simulink model "mrefrobotarm_previous_y_previous_u_previous_ref_cex_3"  (R2018b)
settings: Solver=FixedStepAuto  StartTime=0.0  StopTime=20  RelTol=1e-3  AbsTol=1e-6
undefined symbols (not defined in the file or in its folder): cc, options
libraries: neural x396, simulink x2
(part 11 of 15)

== system mrefrobotarm_previous_y_previous_u_previous_ref_cex_3/cex_m4_10_cl/Layer 3/Delays 1 ==
  "p{3}" : Inport  PortDimensions=30
      mask Display: e = 0.06;c1 = [120 230 180]/255;c2 = ([120 230 180]+0)/(256+128);c3 = ([120 230 180]+128)/(256+128);patch([0 1 1 0],[0 0 1 1],c1);patch([0 1 1 1-e 1-e 0+e],[0 0 1 1-e 0+e 0+e],c2);patch([0 0 1 1-e 0+e 0+e],[0 1 1 1-e 1-e 0+e],c3);plot([0 1 1 0 0],[0 0 1 1 0]);
  mux : Mux  Inputs=1
      mask Display: e = 0.06;c1 = [120 150 230]/255;c2 = ([120 150 230]+0)/383;c3 = ([120 150 230]+128)/383;patch([0 1 1 0],[0 0 1 1],c1);patch([0 1 1 1-e 1-e 0+e],[0 0 1 1-e 0+e 0+e],c2);patch([0 0 1 1-e 0+e 0+e],[0 1 1 1-e 1-e 0+e],c3);plot([0 1 1 0 0],[0 0 1 1 0]);disp('Mux')
  "pd{3,2}" : Outport
      mask Display: e = 0.06;c1 = [120 230 180]/255;c2 = ([120 230 180]+0)/(256+128);c3 = ([120 230 180]+128)/(256+128);patch([0 1 1 0],[0 0 1 1],c1);patch([0 1 1 1-e 1-e 0+e],[0 0 1 1-e 0+e 0+e],c2);patch([0 0 1 1-e 0+e 0+e],[0 1 1 1-e 1-e 0+e],c3);plot([0 1 1 0 0],[0 0 1 1 0]);
  wires:
  "p{3}"/1 -> mux/1
  mux/1 -> "pd{3,2}"/1

== system mrefrobotarm_previous_y_previous_u_previous_ref_cex_3/cex_m4_10_cl/Layer 3/LW{3,2} ==
  "ad{3,2}" : Inport  PortDimensions=30
      mask Display: e = 0.06;c1 = [120 230 180]/255;c2 = ([120 230 180]+0)/(256+128);c3 = ([120 230 180]+128)/(256+128);patch([0 1 1 0],[0 0 1 1],c1);patch([0 1 1 1-e 1-e 0+e],[0 0 1 1-e 0+e 0+e],c2);patch([0 0 1 1-e 0+e 0+e],[0 1 1 1-e 1-e 0+e],c3);plot([0 1 1 0 0],[0 0 1 1 0]);
  "IW{3,2}(1,:)'" : Constant  Value=[-0.022914673180611945524365324899918050505220890045166015625;-0.22416800997145325258230741383158601820468902587890625;0.42578222016399902560834789255750365555286407470703125;-0.1418372366772850667882011066467384807765483856201171875;0.06806813579219629650740586157553480006754398345947265625;-0.26711253758643660471960856739315204322338104248046875;-0.288746492548126509891659452478052116930484771728515625;0.1568382571083110355036893679425702430307865142822265625;-0.1365854357814726416364692340721376240253448486328125;0.86307011627554930388583898093202151358127593994140625;0.314580357392832132834570302293286658823490142822265625;0.056739431746669545530981082492871792055666446685791015625;-0.036816877975223871732879388218862004578113555908203125;-0.04310990977375095400958571190130896866321563720703125;0.1941188152854624870968791583436541259288787841796875;0.2071271857104373947944253586683771573007106781005859375;-0.1944372739173033381998578761340468190610408782958984375;0.47407063712269736921456342315650545060634613037109375;-0.0147826682194927526425853869795901118777692317962646484375;0.01471526546516824067445394774722444708459079265594482421875;0.2010572904622072998304105340139358304440975189208984375;-0.004037117964215650688097891674033235176466405391693115234375;0.254448141541254890807266519914264790713787078857421875;-0.343286635301220222071805210362072102725505828857421875;-0.06292101207340337898354931667199707590043544769287109375;-0.034537508248897015594724990705799427814781665802001953125;0.2287289337043199310972596549618174321949481964111328125;0.472236103182088806651250934010022319853305816650390625;-0.142786618432387102384240051833330653607845306396484375;0.45708708531073305447733901019091717898845672607421875]
      mask Display: e = 0.06;c1 = [120 150 230]/255;c2 = ([120 150 230]+0)/383;c3 = ([120 150 230]+128)/383;patch([0 1 1 0],[0 0 1 1],c1);patch([0 1 1 1-e 1-e 0+e],[0 0 1 1-e 0+e 0+e],c2);patch([0 0 1 1-e 0+e 0+e],[0 1 1 1-e 1-e 0+e],c3);plot([0 1 1 0 0],[0 0 1 1 0]);disp('weights');
  Mux : Mux  Inputs=1
      mask Display: e = 0.06;c1 = [120 150 230]/255;c2 = ([120 150 230]+0)/383;c3 = ([120 150 230]+128)/383;patch([0 1 1 0],[0 0 1 1],c1);patch([0 1 1 1-e 1-e 0+e],[0 0 1 1-e 0+e 0+e],c2);patch([0 0 1 1-e 0+e 0+e],[0 1 1 1-e 1-e 0+e],c3);plot([0 1 1 0 0],[0 0 1 1 0]);disp('Mux');
  dotprod1 : neural/Weight Functions/dotprod
  "lz{3,2}" : Outport
      mask Display: e = 0.06;c1 = [120 230 180]/255;c2 = ([120 230 180]+0)/(256+128);c3 = ([120 230 180]+128)/(256+128);patch([0 1 1 0],[0 0 1 1],c1);patch([0 1 1 1-e 1-e 0+e],[0 0 1 1-e 0+e 0+e],c2);patch([0 0 1 1-e 0+e 0+e],[0 1 1 1-e 1-e 0+e],c3);plot([0 1 1 0 0],[0 0 1 1 0]);
  wires:
  "IW{3,2}(1,:)'"/1 -> dotprod1/1
  "ad{3,2}"/1 -> dotprod1/2
  dotprod1/1 -> Mux/1
  Mux/1 -> "lz{3,2}"/1

== system mrefrobotarm_previous_y_previous_u_previous_ref_cex_3/cex_m5_50/Layer 1/Delays 1 ==
  "p{1}" : Inport  PortDimensions=10
      mask Display: e = 0.06;c1 = [120 230 180]/255;c2 = ([120 230 180]+0)/(256+128);c3 = ([120 230 180]+128)/(256+128);patch([0 1 1 0],[0 0 1 1],c1);patch([0 1 1 1-e 1-e 0+e],[0 0 1 1-e 0+e 0+e],c2);patch([0 0 1 1-e 0+e 0+e],[0 1 1 1-e 1-e 0+e],c3);plot([0 1 1 0 0],[0 0 1 1 0]);
  mux : Mux  Inputs=1
      mask Display: e = 0.06;c1 = [120 150 230]/255;c2 = ([120 150 230]+0)/383;c3 = ([120 150 230]+128)/383;patch([0 1 1 0],[0 0 1 1],c1);patch([0 1 1 1-e 1-e 0+e],[0 0 1 1-e 0+e 0+e],c2);patch([0 0 1 1-e 0+e 0+e],[0 1 1 1-e 1-e 0+e],c3);plot([0 1 1 0 0],[0 0 1 1 0]);disp('Mux')
  "pd{1,1}" : Outport
      mask Display: e = 0.06;c1 = [120 230 180]/255;c2 = ([120 230 180]+0)/(256+128);c3 = ([120 230 180]+128)/(256+128);patch([0 1 1 0],[0 0 1 1],c1);patch([0 1 1 1-e 1-e 0+e],[0 0 1 1-e 0+e 0+e],c2);patch([0 0 1 1-e 0+e 0+e],[0 1 1 1-e 1-e 0+e],c3);plot([0 1 1 0 0],[0 0 1 1 0]);
  wires:
  "p{1}"/1 -> mux/1
  mux/1 -> "pd{1,1}"/1

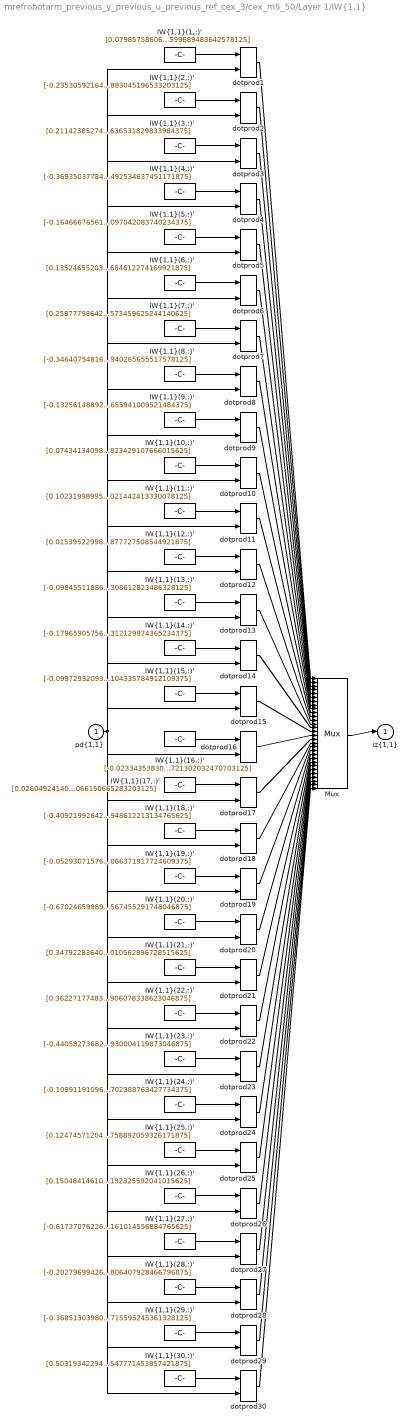
== system mrefrobotarm_previous_y_previous_u_previous_ref_cex_3/cex_m5_50/Layer 1/IW{1,1} ==
  "pd{1,1}" : Inport  PortDimensions=10
      mask Display: e = 0.06;c1 = [120 230 180]/255;c2 = ([120 230 180]+0)/(256+128);c3 = ([120 230 180]+128)/(256+128);patch([0 1 1 0],[0 0 1 1],c1);patch([0 1 1 1-e 1-e 0+e],[0 0 1 1-e 0+e 0+e],c2);patch([0 0 1 1-e 0+e 0+e],[0 1 1 1-e 1-e 0+e],c3);plot([0 1 1 0 0],[0 0 1 1 0]);
  "IW{1,1}(1,:)'" : Constant  Value=[0.079857586064122687563582303482689894735813140869140625;-0.017723095364553236030769056696954066865146160125732421875;-0.056548854768613217303130369373320718295872211456298828125;-0.10470870115022480606459254204310127533972263336181640625;-0.11145776410343340157016456259952974505722522735595703125;-0.040973627042265363396023047926064464263617992401123046875;-0.2352542960460574927861188143651816062629222869873046875;0.074050472634338226907146918165381066501140594482421875;-0.1791921386348343248062775501239229924976825714111328125;0.1353912225675833191917973863382940180599689483642578125]
      mask Display: e = 0.06;c1 = [120 150 230]/255;c2 = ([120 150 230]+0)/383;c3 = ([120 150 230]+128)/383;patch([0 1 1 0],[0 0 1 1],c1);patch([0 1 1 1-e 1-e 0+e],[0 0 1 1-e 0+e 0+e],c2);patch([0 0 1 1-e 0+e 0+e],[0 1 1 1-e 1-e 0+e],c3);plot([0 1 1 0 0],[0 0 1 1 0]);disp('Weights');
  "IW{1,1}(10,:)'" : Constant  Value=[0.0743413409874611463834526148275472223758697509765625;0.164396607140263883994890647954889573156833648681640625;-0.143955487553599936756398847137461416423320770263671875;-0.0721315099709873563949003028028528206050395965576171875;0.1556391323832038986463288665618165396153926849365234375;-0.15582294381245664904866998767829500138759613037109375;0.0193247847981503732828212349659224855713546276092529296875;-0.1039680088534420676626979229695280082523822784423828125;0.08318682925150173990136437396358815021812915802001953125;-0.2231496668480378586796319950735778547823429107666015625]
      mask Display: e = 0.06;c1 = [120 150 230]/255;c2 = ([120 150 230]+0)/383;c3 = ([120 150 230]+128)/383;patch([0 1 1 0],[0 0 1 1],c1);patch([0 1 1 1-e 1-e 0+e],[0 0 1 1-e 0+e 0+e],c2);patch([0 0 1 1-e 0+e 0+e],[0 1 1 1-e 1-e 0+e],c3);plot([0 1 1 0 0],[0 0 1 1 0]);disp('Weights');
  "IW{1,1}(11,:)'" : Constant  Value=[0.102319989954805679044369526309310458600521087646484375;-0.1217472670747620500097951889983960427343845367431640625;0.022250510998612631208271039895407739095389842987060546875;-0.0865197557599649280657416738904430530965328216552734375;0.047157973574144917972006396666984073817729949951171875;0.166311308504842270128420977925998158752918243408203125;-0.07692919866478746537818977913048001937568187713623046875;0.1289101580164291604990722817092319019138813018798828125;-0.03712492046256300748385825727382325567305088043212890625;0.0862830620540880055546750782013987191021442413330078125]
      mask Display: e = 0.06;c1 = [120 150 230]/255;c2 = ([120 150 230]+0)/383;c3 = ([120 150 230]+128)/383;patch([0 1 1 0],[0 0 1 1],c1);patch([0 1 1 1-e 1-e 0+e],[0 0 1 1-e 0+e 0+e],c2);patch([0 0 1 1-e 0+e 0+e],[0 1 1 1-e 1-e 0+e],c3);plot([0 1 1 0 0],[0 0 1 1 0]);disp('Weights');
  "IW{1,1}(12,:)'" : Constant  Value=[0.0153952299864565760045831410707251052372157573699951171875;-0.29382621968364486253477707577985711395740509033203125;0.15069864020460455034111646455130539834499359130859375;0.129272775534195083491084687921102158725261688232421875;-0.00719280555420370899810666998064334620721638202667236328125;0.017590441101808795831829002054291777312755584716796875;-0.1455726439346946843311769725914928130805492401123046875;-0.1131091311033599888791201237836503423750400543212890625;0.144361291612564779374139334322535432875156402587890625;-0.1039940199905408924063721087804879061877727508544921875]
      mask Display: e = 0.06;c1 = [120 150 230]/255;c2 = ([120 150 230]+0)/383;c3 = ([120 150 230]+128)/383;patch([0 1 1 0],[0 0 1 1],c1);patch([0 1 1 1-e 1-e 0+e],[0 0 1 1-e 0+e 0+e],c2);patch([0 0 1 1-e 0+e 0+e],[0 1 1 1-e 1-e 0+e],c3);plot([0 1 1 0 0],[0 0 1 1 0]);disp('Weights');
  "IW{1,1}(13,:)'" : Constant  Value=[-0.09845511886806544710193378477924852631986141204833984375;0.09093880387205426074626046784032951109111309051513671875;-0.00807145029070374143975730163447224185802042484283447265625;0.1579263851539709495597207933315075933933258056640625;-0.0894690058866917381497074757135123945772647857666015625;-0.0062623475836107826697496392398534226231276988983154296875;0.06411970043190341750349858784829848445951938629150390625;-0.11454387947590256857655077737945248372852802276611328125;-0.16589537965291556442792852976708672940731048583984375;0.197603240212231856531843732227571308612823486328125]
      mask Display: e = 0.06;c1 = [120 150 230]/255;c2 = ([120 150 230]+0)/383;c3 = ([120 150 230]+128)/383;patch([0 1 1 0],[0 0 1 1],c1);patch([0 1 1 1-e 1-e 0+e],[0 0 1 1-e 0+e 0+e],c2);patch([0 0 1 1-e 0+e 0+e],[0 1 1 1-e 1-e 0+e],c3);plot([0 1 1 0 0],[0 0 1 1 0]);disp('Weights');
  "IW{1,1}(14,:)'" : Constant  Value=[-0.1796590575681936419183415409861481748521327972412109375;0.004065668616646420270577255706712094251997768878936767578125;0.1660524217557300674652509542283951304852962493896484375;-0.018752259357130311723249604938246193341910839080810546875;-0.0166360990303930332545601089577758102677762508392333984375;0.156250719589604736281529540065093897283077239990234375;0.143670141139804530272527927081682719290256500244140625;0.197765834991741107362628326882258988916873931884765625;-0.115318383987298600512616530977538786828517913818359375;0.06920828841457514479795776196624501608312129974365234375]
      mask Display: e = 0.06;c1 = [120 150 230]/255;c2 = ([120 150 230]+0)/383;c3 = ([120 150 230]+128)/383;patch([0 1 1 0],[0 0 1 1],c1);patch([0 1 1 1-e 1-e 0+e],[0 0 1 1-e 0+e 0+e],c2);patch([0 0 1 1-e 0+e 0+e],[0 1 1 1-e 1-e 0+e],c3);plot([0 1 1 0 0],[0 0 1 1 0]);disp('Weights');
  "IW{1,1}(15,:)'" : Constant  Value=[-0.0997293209396606095129556024403427727520465850830078125;-0.220637160043276825405200725072063505649566650390625;-0.00148221978238747219801252352766596231958828866481781005859375;-0.2518385145644688183352855048724450170993804931640625;-0.226371647407521858763601585451397113502025604248046875;-0.183592461943430762527640354164759628474712371826171875;-0.0281470738205235916640223337026327499188482761383056640625;-0.183673166456358061271458836927195079624652862548828125;0.03735748593921994764599503469071350991725921630859375;-0.083966000578261590359119281856692396104335784912109375]
      mask Display: e = 0.06;c1 = [120 150 230]/255;c2 = ([120 150 230]+0)/383;c3 = ([120 150 230]+128)/383;patch([0 1 1 0],[0 0 1 1],c1);patch([0 1 1 1-e 1-e 0+e],[0 0 1 1-e 0+e 0+e],c2);patch([0 0 1 1-e 0+e 0+e],[0 1 1 1-e 1-e 0+e],c3);plot([0 1 1 0 0],[0 0 1 1 0]);disp('Weights');
  "IW{1,1}(16,:)'" : Constant  Value=[-0.023343538302298010023161367598731885664165019989013671875;0.207808437401322265714043169282376766204833984375;0.19767903767718764118654917183448560535907745361328125;0.08721736450330919154794173664413392543792724609375;-0.1026675757733719607234235127179999835789203643798828125;0.1893806324687653253047159296329482458531856536865234375;0.157181246537321739342729642885387875139713287353515625;-0.0762455615664333341552350020720041356980800628662109375;0.1511383886935200038248439113885979168117046356201171875;-0.032936019457746275318488216043988359160721302032470703125]
      mask Display: e = 0.06;c1 = [120 150 230]/255;c2 = ([120 150 230]+0)/383;c3 = ([120 150 230]+128)/383;patch([0 1 1 0],[0 0 1 1],c1);patch([0 1 1 1-e 1-e 0+e],[0 0 1 1-e 0+e 0+e],c2);patch([0 0 1 1-e 0+e 0+e],[0 1 1 1-e 1-e 0+e],c3);plot([0 1 1 0 0],[0 0 1 1 0]);disp('Weights');
  "IW{1,1}(17,:)'" : Constant  Value=[0.026049241400837468141116204378704424016177654266357421875;-0.032936276559719333822950915191540843807160854339599609375;-0.09167093550109205180032034832038334570825099945068359375;-0.1285074909294273981519296512487926520407199859619140625;0.078280680856052831106950407047406770288944244384765625;0.035046276117616514955699358324636705219745635986328125;0.04575276258096482029369411748120910488069057464599609375;-0.1455865211885374044253893544009770266711711883544921875;-0.16108537419119872691197770109283737838268280029296875;-0.25221969637927810214961255041998811066150665283203125]
      mask Display: e = 0.06;c1 = [120 150 230]/255;c2 = ([120 150 230]+0)/383;c3 = ([120 150 230]+128)/383;patch([0 1 1 0],[0 0 1 1],c1);patch([0 1 1 1-e 1-e 0+e],[0 0 1 1-e 0+e 0+e],c2);patch([0 0 1 1-e 0+e 0+e],[0 1 1 1-e 1-e 0+e],c3);plot([0 1 1 0 0],[0 0 1 1 0]);disp('Weights');
  "IW{1,1}(18,:)'" : Constant  Value=[-0.409219926426756586135269344595144502818584442138671875;0.0785959772336427830996541388230980373919010162353515625;-0.150796017332621434814399208335089497268199920654296875;0.054714100522777205093394314872057293541729450225830078125;-0.197699818473965283072146803533541969954967498779296875;0.079927612600015407462450411912868730723857879638671875;0.0100629098409829621785238629172454238869249820709228515625;-0.2085223358752021083351024799412698484957218170166015625;0.1160915267315043575280242293956689536571502685546875;-0.039902292098272375275858081522528664208948612213134765625]
      mask Display: e = 0.06;c1 = [120 150 230]/255;c2 = ([120 150 230]+0)/383;c3 = ([120 150 230]+128)/383;patch([0 1 1 0],[0 0 1 1],c1);patch([0 1 1 1-e 1-e 0+e],[0 0 1 1-e 0+e 0+e],c2);patch([0 0 1 1-e 0+e 0+e],[0 1 1 1-e 1-e 0+e],c3);plot([0 1 1 0 0],[0 0 1 1 0]);disp('Weights');
  "IW{1,1}(19,:)'" : Constant  Value=[-0.05293071576668927080699944553998648189008235931396484375;-0.0784315336245811345339262743436847813427448272705078125;0.052396564711746758391530676135516841895878314971923828125;-0.045966369293603072387899288742119097150862216949462890625;0.1996321210973512894071291157160885632038116455078125;-0.047923892413621015096136801503234892152249813079833984375;0.250968980826343390777566355609451420605182647705078125;0.0226665665494998093409950712384670623578131198883056640625;-0.1273645483236649778024940360410255379974842071533203125;-0.0881084613766523749855963387744850479066371917724609375]
      mask Display: e = 0.06;c1 = [120 150 230]/255;c2 = ([120 150 230]+0)/383;c3 = ([120 150 230]+128)/383;patch([0 1 1 0],[0 0 1 1],c1);patch([0 1 1 1-e 1-e 0+e],[0 0 1 1-e 0+e 0+e],c2);patch([0 0 1 1-e 0+e 0+e],[0 1 1 1-e 1-e 0+e],c3);plot([0 1 1 0 0],[0 0 1 1 0]);disp('Weights');
  "IW{1,1}(2,:)'" : Constant  Value=[-0.2353059216442040246786149282343103550374507904052734375;-0.37789763749456184438457739815930835902690887451171875;0.214493078021647687325668130142730660736560821533203125;0.130691057428845069932066280671278946101665496826171875;0.192062118999956565890130377738387323915958404541015625;0.09267188455379683775792187816477962769567966461181640625;0.04144170290809519319186193797577288933098316192626953125;-0.016488872173757489203449466685924562625586986541748046875;-0.411465202425676135344900785639765672385692596435546875;0.1802654075409109435401688870115322060883045196533203125]
      mask Display: e = 0.06;c1 = [120 150 230]/255;c2 = ([120 150 230]+0)/383;c3 = ([120 150 230]+128)/383;patch([0 1 1 0],[0 0 1 1],c1);patch([0 1 1 1-e 1-e 0+e],[0 0 1 1-e 0+e 0+e],c2);patch([0 0 1 1-e 0+e 0+e],[0 1 1 1-e 1-e 0+e],c3);plot([0 1 1 0 0],[0 0 1 1 0]);disp('Weights');
  "IW{1,1}(20,:)'" : Constant  Value=[-0.670246599899003481226600342779420316219329833984375;0.54023279823907544017203008479555137455463409423828125;-0.132643633303448360560850005640531890094280242919921875;-0.08573477507453254597979963591569685377180576324462890625;-0.05214787663669749606665249075376777909696102142333984375;-0.24868608156944926879106105843675322830677032470703125;-0.0708532779744801555210642618476413190364837646484375;-0.1612321158738975468427412351957173086702823638916015625;-0.377010414829936857383785309139057062566280364990234375;-0.326354942562080363455123688254388980567455291748046875]
      mask Display: e = 0.06;c1 = [120 150 230]/255;c2 = ([120 150 230]+0)/383;c3 = ([120 150 230]+128)/383;patch([0 1 1 0],[0 0 1 1],c1);patch([0 1 1 1-e 1-e 0+e],[0 0 1 1-e 0+e 0+e],c2);patch([0 0 1 1-e 0+e 0+e],[0 1 1 1-e 1-e 0+e],c3);plot([0 1 1 0 0],[0 0 1 1 0]);disp('Weights');
  "IW{1,1}(21,:)'" : Constant  Value=[0.34792283640337806627229610967333428561687469482421875;0.052295351768964971894693150034072459675371646881103515625;0.215517399724929281656926605137414298951625823974609375;-0.10110471240800637804380102124923723749816417694091796875;-0.1307353664929510606018681073692278005182743072509765625;0.152266018278392090135042735710158012807369232177734375;-0.149298402696842857917403080136864446103572845458984375;0.044436751362071459647840043771793716587126255035400390625;0.256340040153919812571103875598055310547351837158203125;0.05083490551971847626333556036115624010562896728515625]
      mask Display: e = 0.06;c1 = [120 150 230]/255;c2 = ([120 150 230]+0)/383;c3 = ([120 150 230]+128)/383;patch([0 1 1 0],[0 0 1 1],c1);patch([0 1 1 1-e 1-e 0+e],[0 0 1 1-e 0+e 0+e],c2);patch([0 0 1 1-e 0+e 0+e],[0 1 1 1-e 1-e 0+e],c3);plot([0 1 1 0 0],[0 0 1 1 0]);disp('Weights');
  "IW{1,1}(22,:)'" : Constant  Value=[0.362271774839149018898609710959135554730892181396484375;-0.1319520713686885837745421667932532727718353271484375;-0.1014321707030214347877716818402404896914958953857421875;-0.09152058110484677377893802940889145247638225555419921875;-0.0042955190046048523366817306623488548211753368377685546875;0.01111324222692758496855436334271871601231396198272705078125;0.1775136539958918902026852038034121505916118621826171875;-0.0521229797522363147432855612350977025926113128662109375;0.11161762706013632351353948024552664719521999359130859375;0.36427552672722807169947145666810683906078338623046875]
      mask Display: e = 0.06;c1 = [120 150 230]/255;c2 = ([120 150 230]+0)/383;c3 = ([120 150 230]+128)/383;patch([0 1 1 0],[0 0 1 1],c1);patch([0 1 1 1-e 1-e 0+e],[0 0 1 1-e 0+e 0+e],c2);patch([0 0 1 1-e 0+e 0+e],[0 1 1 1-e 1-e 0+e],c3);plot([0 1 1 0 0],[0 0 1 1 0]);disp('Weights');
  "IW{1,1}(23,:)'" : Constant  Value=[-0.440582736828079968294247237281524576246738433837890625;0.062056781177113336245287911197010544128715991973876953125;0.06482205563836225536977764249968458898365497589111328125;0.125994684923841304691194409315357916057109832763671875;0.20426644517248504495654515267233364284038543701171875;0.0263028477064109512950640379358446807600557804107666015625;-0.0263181703085152325638507164740076404996216297149658203125;-0.038622682868921433263498244059519493021070957183837890625;0.11278063952137755421301079650220344774425029754638671875;-0.2220891765070327206199607417147490195930004119873046875]
      mask Display: e = 0.06;c1 = [120 150 230]/255;c2 = ([120 150 230]+0)/383;c3 = ([120 150 230]+128)/383;patch([0 1 1 0],[0 0 1 1],c1);patch([0 1 1 1-e 1-e 0+e],[0 0 1 1-e 0+e 0+e],c2);patch([0 0 1 1-e 0+e 0+e],[0 1 1 1-e 1-e 0+e],c3);plot([0 1 1 0 0],[0 0 1 1 0]);disp('Weights');
  "IW{1,1}(24,:)'" : Constant  Value=[-0.1099119109681839512315804086028947494924068450927734375;0.1508099505426872821711725691784522496163845062255859375;-0.12041229586109179761077569992266944609582424163818359375;0.25238005086023751477597443226841278374195098876953125;0.11438877306951240886423448728237417526543140411376953125;0.2137468471614491216659104111386113800108432769775390625;0.11488748725941888562118720074067823588848114013671875;0.060073228498920487605783335993692162446677684783935546875;0.0659200601810043529393823291684384457767009735107421875;0.10255176189659041818824647407382144592702388763427734375]
      mask Display: e = 0.06;c1 = [120 150 230]/255;c2 = ([120 150 230]+0)/383;c3 = ([120 150 230]+128)/383;patch([0 1 1 0],[0 0 1 1],c1);patch([0 1 1 1-e 1-e 0+e],[0 0 1 1-e 0+e 0+e],c2);patch([0 0 1 1-e 0+e 0+e],[0 1 1 1-e 1-e 0+e],c3);plot([0 1 1 0 0],[0 0 1 1 0]);disp('Weights');
  "IW{1,1}(25,:)'" : Constant  Value=[0.1247457120471533176253586816528695635497570037841796875;0.08475288443967875229301256467806524597108364105224609375;0.150738537226991431428047008012072183191776275634765625;-0.039317157200356056545587080108816735446453094482421875;-0.15825890037866552351175641888403333723545074462890625;0.10080224229780039568726834886547294445335865020751953125;-0.03808289855491621411776037575691589154303073883056640625;0.189319003610914304847057110237074084579944610595703125;0.1432633330570446672513895691736252047121524810791015625;-0.1480683003937994512977383010365883819758892059326171875]
      mask Display: e = 0.06;c1 = [120 150 230]/255;c2 = ([120 150 230]+0)/383;c3 = ([120 150 230]+128)/383;patch([0 1 1 0],[0 0 1 1],c1);patch([0 1 1 1-e 1-e 0+e],[0 0 1 1-e 0+e 0+e],c2);patch([0 0 1 1-e 0+e 0+e],[0 1 1 1-e 1-e 0+e],c3);plot([0 1 1 0 0],[0 0 1 1 0]);disp('Weights');
  "IW{1,1}(26,:)'" : Constant  Value=[0.1504841461069787167392775018015527166426181793212890625;0.1706761854885774087886574079675483517348766326904296875;-0.12315763767946487361459873000057996250689029693603515625;-0.105454216674881029458532566422945819795131683349609375;0.079583904076185818521338433129130862653255462646484375;0.083020649045482619587943418082431890070438385009765625;0.1803413532371868355230759561891318298876285552978515625;0.044235880069422826854630415027713752351701259613037109375;0.0303549133863007976341652494056688738055527210235595703125;-0.006131225040918280612400881324219881207682192325592041015625]
      mask Display: e = 0.06;c1 = [120 150 230]/255;c2 = ([120 150 230]+0)/383;c3 = ([120 150 230]+128)/383;patch([0 1 1 0],[0 0 1 1],c1);patch([0 1 1 1-e 1-e 0+e],[0 0 1 1-e 0+e 0+e],c2);patch([0 0 1 1-e 0+e 0+e],[0 1 1 1-e 1-e 0+e],c3);plot([0 1 1 0 0],[0 0 1 1 0]);disp('Weights');
  "IW{1,1}(27,:)'" : Constant  Value=[-0.6173707622614739154442986546200700104236602783203125;0.1739730823776983459350020666533964686095714569091796875;-0.18779220945027630396140239099622704088687896728515625;-0.189501484652068008518455144439940340816974639892578125;-0.0778438999445635604335080870441743172705173492431640625;-0.036877440154400718819172055873423232696950435638427734375;0.1391205346786328345132233152980916202068328857421875;0.12395529611598998798172033275477588176727294921875;0.0122518582229891974388902298187531414441764354705810546875;-0.16963550703672203301408671904937364161014556884765625]
      mask Display: e = 0.06;c1 = [120 150 230]/255;c2 = ([120 150 230]+0)/383;c3 = ([120 150 230]+128)/383;patch([0 1 1 0],[0 0 1 1],c1);patch([0 1 1 1-e 1-e 0+e],[0 0 1 1-e 0+e 0+e],c2);patch([0 0 1 1-e 0+e 0+e],[0 1 1 1-e 1-e 0+e],c3);plot([0 1 1 0 0],[0 0 1 1 0]);disp('Weights');
  "IW{1,1}(28,:)'" : Constant  Value=[-0.2027969942616466847429279596326523460447788238525390625;0.09449207799621735237582953459423151798546314239501953125;0.10270026220038541708845514222048223018646240234375;0.0131710480805120010161513022239887504838407039642333984375;0.1003675370796837940101653430247097276151180267333984375;-0.103832866146567337484185600260389037430286407470703125;-0.07789077517837526831723238274207687936723232269287109375;0.11386227011921858098819626547992811538279056549072265625;0.1150130827350047957313705637716338969767093658447265625;-0.03748247067678149579972313176767784170806407928466796875]
      mask Display: e = 0.06;c1 = [120 150 230]/255;c2 = ([120 150 230]+0)/383;c3 = ([120 150 230]+128)/383;patch([0 1 1 0],[0 0 1 1],c1);patch([0 1 1 1-e 1-e 0+e],[0 0 1 1-e 0+e 0+e],c2);patch([0 0 1 1-e 0+e 0+e],[0 1 1 1-e 1-e 0+e],c3);plot([0 1 1 0 0],[0 0 1 1 0]);disp('Weights');
  "IW{1,1}(29,:)'" : Constant  Value=[-0.36851303980232119616999852951266802847385406494140625;-0.09920798849380034478695478128429385833442211151123046875;0.0037578359588317611188201805560993307153694331645965576171875;-0.1238776540164794603970932485026423819363117218017578125;0.10176668715865055947489281606976874172687530517578125;-0.1272210541501615221893217722026747651398181915283203125;-0.06597747730321346093518286579637788236141204833984375;-0.16785280049088158182968300025095231831073760986328125;-0.2407709885528765691997676867686095647513866424560546875;0.07551578438714785790342176596823264844715595245361328125]
      mask Display: e = 0.06;c1 = [120 150 230]/255;c2 = ([120 150 230]+0)/383;c3 = ([120 150 230]+128)/383;patch([0 1 1 0],[0 0 1 1],c1);patch([0 1 1 1-e 1-e 0+e],[0 0 1 1-e 0+e 0+e],c2);patch([0 0 1 1-e 0+e 0+e],[0 1 1 1-e 1-e 0+e],c3);plot([0 1 1 0 0],[0 0 1 1 0]);disp('Weights');
  "IW{1,1}(3,:)'" : Constant  Value=[0.211423652744485102150662214626208879053592681884765625;0.13742873712692615928432360306032933294773101806640625;0.1351370590578790664704200708001735620200634002685546875;0.222924965995400292673167541579459793865680694580078125;0.2146756433420459464489482570570544339716434478759765625;0.1301919312676363682523827947079553268849849700927734375;0.113146063465918433887935634629684500396251678466796875;0.1425404118328864877529582599891000427305698394775390625;0.0834948087549631512427339430360007099807262420654296875;0.0845220331684256309667802042895345948636531829833984375]
      mask Display: e = 0.06;c1 = [120 150 230]/255;c2 = ([120 150 230]+0)/383;c3 = ([120 150 230]+128)/383;patch([0 1 1 0],[0 0 1 1],c1);patch([0 1 1 1-e 1-e 0+e],[0 0 1 1-e 0+e 0+e],c2);patch([0 0 1 1-e 0+e 0+e],[0 1 1 1-e 1-e 0+e],c3);plot([0 1 1 0 0],[0 0 1 1 0]);disp('Weights');
  "IW{1,1}(30,:)'" : Constant  Value=[0.50319342294712054997063432892900891602039337158203125;0.1347134435099232308008510017316439189016819000244140625;0.01987678330226982925665879520238377153873443603515625;0.1480613773388992637780603445207816548645496368408203125;0.0248397824064196803828252768653328530490398406982421875;-0.1047635853561354746243949875861289910972118377685546875;-0.049682783963678235628069757012781337834894657135009765625;-0.100735025400120747907095619666506536304950714111328125;0.1655564021551410025523409785819239914417266845703125;0.27345997939707522572660991500015370547771453857421875]
      mask Display: e = 0.06;c1 = [120 150 230]/255;c2 = ([120 150 230]+0)/383;c3 = ([120 150 230]+128)/383;patch([0 1 1 0],[0 0 1 1],c1);patch([0 1 1 1-e 1-e 0+e],[0 0 1 1-e 0+e 0+e],c2);patch([0 0 1 1-e 0+e 0+e],[0 1 1 1-e 1-e 0+e],c3);plot([0 1 1 0 0],[0 0 1 1 0]);disp('Weights');
  "IW{1,1}(4,:)'" : Constant  Value=[-0.3693503778477615906439268655958585441112518310546875;-0.67122941808021863163702391830156557261943817138671875;0.1111473382234235696142121696539106778800487518310546875;-0.040736390935827836157212544776484719477593898773193359375;-0.0353356023442425171143810302964993752539157867431640625;0.01216229985190520578031136977870119153521955013275146484375;-0.10404525704894747317741376946287346072494983673095703125;-0.104780197789657913975958081209682859480381011962890625;-0.53806327163552813974689570386544801294803619384765625;0.05700246094633869275991600034103612415492534637451171875]
      mask Display: e = 0.06;c1 = [120 150 230]/255;c2 = ([120 150 230]+0)/383;c3 = ([120 150 230]+128)/383;patch([0 1 1 0],[0 0 1 1],c1);patch([0 1 1 1-e 1-e 0+e],[0 0 1 1-e 0+e 0+e],c2);patch([0 0 1 1-e 0+e 0+e],[0 1 1 1-e 1-e 0+e],c3);plot([0 1 1 0 0],[0 0 1 1 0]);disp('Weights');
  "IW{1,1}(5,:)'" : Constant  Value=[-0.164666765612599963475304321036674082279205322265625;-0.0998422856616774934135349894859245978295803070068359375;-0.09462503298437634213780000891347299329936504364013671875;0.03430917193931425079878039241521037183701992034912109375;-0.03477462302654032999527089486946351826190948486328125;0.032130815971161456878757434196813846938312053680419921875;-0.1379698668978186770761595880685490556061267852783203125;-0.15709713424736604370224313242943026125431060791015625;0.13296358161434962408264937039348296821117401123046875;-0.09362976472028582131112983688581152819097042083740234375]
      mask Display: e = 0.06;c1 = [120 150 230]/255;c2 = ([120 150 230]+0)/383;c3 = ([120 150 230]+128)/383;patch([0 1 1 0],[0 0 1 1],c1);patch([0 1 1 1-e 1-e 0+e],[0 0 1 1-e 0+e 0+e],c2);patch([0 0 1 1-e 0+e 0+e],[0 1 1 1-e 1-e 0+e],c3);plot([0 1 1 0 0],[0 0 1 1 0]);disp('Weights');
  "IW{1,1}(6,:)'" : Constant  Value=[0.1352465520388095310266862725256942212581634521484375;0.0214581692328368288380513462243470712564885616302490234375;0.10411609803656819706052516494310111738741397857666015625;-0.1575814292668583360690348627031198702752590179443359375;0.1337643139091573007970481512529659084975719451904296875;-0.09826198783057456254130812567382236011326313018798828125;-0.148171383911512910547259025406674481928348541259765625;-0.0210561242976584801767092613999921013601124286651611328125;-0.049158108380956973271214138776485924609005451202392578125;0.076438612259305649399010462730075232684612274169921875]
      mask Display: e = 0.06;c1 = [120 150 230]/255;c2 = ([120 150 230]+0)/383;c3 = ([120 150 230]+128)/383;patch([0 1 1 0],[0 0 1 1],c1);patch([0 1 1 1-e 1-e 0+e],[0 0 1 1-e 0+e 0+e],c2);patch([0 0 1 1-e 0+e 0+e],[0 1 1 1-e 1-e 0+e],c3);plot([0 1 1 0 0],[0 0 1 1 0]);disp('Weights');
  "IW{1,1}(7,:)'" : Constant  Value=[0.25877798642947469343056354773580096662044525146484375;-0.1347552537880535028502748673417954705655574798583984375;0.2230600448704475879946329541780869476497173309326171875;0.12369687977622813301881166125895106233656406402587890625;0.0175991040708676736714632937719215988181531429290771484375;0.03244132342467694052334792331748758442699909210205078125;0.053287446651061394498061218882867251522839069366455078125;0.1679503255953132268007976790613611228764057159423828125;-0.011092710773502094390163819070949102751910686492919921875;0.287440145752466735817876042347052134573459625244140625]
      mask Display: e = 0.06;c1 = [120 150 230]/255;c2 = ([120 150 230]+0)/383;c3 = ([120 150 230]+128)/383;patch([0 1 1 0],[0 0 1 1],c1);patch([0 1 1 1-e 1-e 0+e],[0 0 1 1-e 0+e 0+e],c2);patch([0 0 1 1-e 0+e 0+e],[0 1 1 1-e 1-e 0+e],c3);plot([0 1 1 0 0],[0 0 1 1 0]);disp('Weights');
  "IW{1,1}(8,:)'" : Constant  Value=[-0.346407548164190670636486402145237661898136138916015625;-0.046465774203113742457649237849182100035250186920166015625;-0.2086198841595223452127783048126730136573314666748046875;-0.1493474983814212231347795523106469772756099700927734375;0.029068484144803556634695240745713817887008190155029296875;-0.151664488848971157342049309590947814285755157470703125;0.098074934235973909579797691549174487590789794921875;0.09897481812097612408063440625483053736388683319091796875;-0.1395660439653094997414228828347404487431049346923828125;-0.11713029802466856654774574053590185940265655517578125]
      mask Display: e = 0.06;c1 = [120 150 230]/255;c2 = ([120 150 230]+0)/383;c3 = ([120 150 230]+128)/383;patch([0 1 1 0],[0 0 1 1],c1);patch([0 1 1 1-e 1-e 0+e],[0 0 1 1-e 0+e 0+e],c2);patch([0 0 1 1-e 0+e 0+e],[0 1 1 1-e 1-e 0+e],c3);plot([0 1 1 0 0],[0 0 1 1 0]);disp('Weights');
  "IW{1,1}(9,:)'" : Constant  Value=[-0.1325614889291009956817646298077306710183620452880859375;-0.114098108150274935024270916983368806540966033935546875;-0.0110703317849722392141043059154981165193021297454833984375;0.08305659374215380863493152219234616495668888092041015625;0.038164246669630530472971940980642102658748626708984375;-0.0105523024232770656904989436952746473252773284912109375;-0.19323700741089855359433613557484932243824005126953125;0.260491238401214963982255312657798640429973602294921875;0.0427307156404077570499566718353889882564544677734375;0.01355718185507891193619656178270815871655941009521484375]
      mask Display: e = 0.06;c1 = [120 150 230]/255;c2 = ([120 150 230]+0)/383;c3 = ([120 150 230]+128)/383;patch([0 1 1 0],[0 0 1 1],c1);patch([0 1 1 1-e 1-e 0+e],[0 0 1 1-e 0+e 0+e],c2);patch([0 0 1 1-e 0+e 0+e],[0 1 1 1-e 1-e 0+e],c3);plot([0 1 1 0 0],[0 0 1 1 0]);disp('Weights');
  Mux : Mux  Inputs=30
      mask Display: e = 0.06;c1 = [120 150 230]/255;c2 = ([120 150 230]+0)/383;c3 = ([120 150 230]+128)/383;patch([0 1 1 0],[0 0 1 1],c1);patch([0 1 1 1-e 1-e 0+e],[0 0 1 1-e 0+e 0+e],c2);patch([0 0 1 1-e 0+e 0+e],[0 1 1 1-e 1-e 0+e],c3);plot([0 1 1 0 0],[0 0 1 1 0]);disp('Mux');
  dotprod{1..30} (30 alike) : neural/Weight Functions/dotprod
  "iz{1,1}" : Outport
      mask Display: e = 0.06;c1 = [120 230 180]/255;c2 = ([120 230 180]+0)/(256+128);c3 = ([120 230 180]+128)/(256+128);patch([0 1 1 0],[0 0 1 1],c1);patch([0 1 1 1-e 1-e 0+e],[0 0 1 1-e 0+e 0+e],c2);patch([0 0 1 1-e 0+e 0+e],[0 1 1 1-e 1-e 0+e],c3);plot([0 1 1 0 0],[0 0 1 1 0]);
  wires:
  "IW{1,1}(1,:)'"/1 -> dotprod1/1
  "pd{1,1}"/1 -> dotprod1/2, dotprod2/2, dotprod3/2, dotprod4/2, dotprod5/2, dotprod6/2, dotprod7/2, dotprod8/2, dotprod9/2, dotprod10/2, dotprod11/2, dotprod12/2, dotprod13/2, dotprod14/2, dotprod15/2, dotprod16/2, dotprod17/2, dotprod18/2, dotprod19/2, dotprod20/2, dotprod21/2, dotprod22/2, dotprod23/2, dotprod24/2, dotprod25/2, dotprod26/2, dotprod27/2, dotprod28/2, dotprod29/2, dotprod30/2
  dotprod1/1 -> Mux/1
  "IW{1,1}(2,:)'"/1 -> dotprod2/1
  dotprod2/1 -> Mux/2
  "IW{1,1}(3,:)'"/1 -> dotprod3/1
  dotprod3/1 -> Mux/3
  "IW{1,1}(4,:)'"/1 -> dotprod4/1
  dotprod4/1 -> Mux/4
  "IW{1,1}(5,:)'"/1 -> dotprod5/1
  dotprod5/1 -> Mux/5
  "IW{1,1}(6,:)'"/1 -> dotprod6/1
  dotprod6/1 -> Mux/6
  "IW{1,1}(7,:)'"/1 -> dotprod7/1
  dotprod7/1 -> Mux/7
  "IW{1,1}(8,:)'"/1 -> dotprod8/1
  dotprod8/1 -> Mux/8
  "IW{1,1}(9,:)'"/1 -> dotprod9/1
  dotprod9/1 -> Mux/9
  "IW{1,1}(10,:)'"/1 -> dotprod10/1
  dotprod10/1 -> Mux/10
  "IW{1,1}(11,:)'"/1 -> dotprod11/1
  dotprod11/1 -> Mux/11
  "IW{1,1}(12,:)'"/1 -> dotprod12/1
  dotprod12/1 -> Mux/12
  "IW{1,1}(13,:)'"/1 -> dotprod13/1
  dotprod13/1 -> Mux/13
  "IW{1,1}(14,:)'"/1 -> dotprod14/1
  dotprod14/1 -> Mux/14
  "IW{1,1}(15,:)'"/1 -> dotprod15/1
  dotprod15/1 -> Mux/15
  "IW{1,1}(16,:)'"/1 -> dotprod16/1
  dotprod16/1 -> Mux/16
  "IW{1,1}(17,:)'"/1 -> dotprod17/1
  dotprod17/1 -> Mux/17
  "IW{1,1}(18,:)'"/1 -> dotprod18/1
  dotprod18/1 -> Mux/18
  "IW{1,1}(19,:)'"/1 -> dotprod19/1
  dotprod19/1 -> Mux/19
  "IW{1,1}(20,:)'"/1 -> dotprod20/1
  dotprod20/1 -> Mux/20
  "IW{1,1}(21,:)'"/1 -> dotprod21/1
  dotprod21/1 -> Mux/21
  "IW{1,1}(22,:)'"/1 -> dotprod22/1
  dotprod22/1 -> Mux/22
  "IW{1,1}(23,:)'"/1 -> dotprod23/1
  dotprod23/1 -> Mux/23
  "IW{1,1}(24,:)'"/1 -> dotprod24/1
  dotprod24/1 -> Mux/24
  "IW{1,1}(25,:)'"/1 -> dotprod25/1
  dotprod25/1 -> Mux/25
  "IW{1,1}(26,:)'"/1 -> dotprod26/1
  dotprod26/1 -> Mux/26
  "IW{1,1}(27,:)'"/1 -> dotprod27/1
  dotprod27/1 -> Mux/27
  "IW{1,1}(28,:)'"/1 -> dotprod28/1
  dotprod28/1 -> Mux/28
  "IW{1,1}(29,:)'"/1 -> dotprod29/1
  dotprod29/1 -> Mux/29
  "IW{1,1}(30,:)'"/1 -> dotprod30/1
  dotprod30/1 -> Mux/30
  Mux/1 -> "iz{1,1}"/1

== system mrefrobotarm_previous_y_previous_u_previous_ref_cex_3/cex_m5_50/Layer 2/Delays 1 ==
  "p{2}" : Inport  PortDimensions=30
      mask Display: e = 0.06;c1 = [120 230 180]/255;c2 = ([120 230 180]+0)/(256+128);c3 = ([120 230 180]+128)/(256+128);patch([0 1 1 0],[0 0 1 1],c1);patch([0 1 1 1-e 1-e 0+e],[0 0 1 1-e 0+e 0+e],c2);patch([0 0 1 1-e 0+e 0+e],[0 1 1 1-e 1-e 0+e],c3);plot([0 1 1 0 0],[0 0 1 1 0]);
  mux : Mux  Inputs=1
      mask Display: e = 0.06;c1 = [120 150 230]/255;c2 = ([120 150 230]+0)/383;c3 = ([120 150 230]+128)/383;patch([0 1 1 0],[0 0 1 1],c1);patch([0 1 1 1-e 1-e 0+e],[0 0 1 1-e 0+e 0+e],c2);patch([0 0 1 1-e 0+e 0+e],[0 1 1 1-e 1-e 0+e],c3);plot([0 1 1 0 0],[0 0 1 1 0]);disp('Mux')
  "pd{2,1}" : Outport
      mask Display: e = 0.06;c1 = [120 230 180]/255;c2 = ([120 230 180]+0)/(256+128);c3 = ([120 230 180]+128)/(256+128);patch([0 1 1 0],[0 0 1 1],c1);patch([0 1 1 1-e 1-e 0+e],[0 0 1 1-e 0+e 0+e],c2);patch([0 0 1 1-e 0+e 0+e],[0 1 1 1-e 1-e 0+e],c3);plot([0 1 1 0 0],[0 0 1 1 0]);
  wires:
  "p{2}"/1 -> mux/1
  mux/1 -> "pd{2,1}"/1
